simulink model "sedemo_event_translation_delay"  (Simulink 7.5)
settings: Solver=VariableStepDiscrete  StartTime=0.0  StopTime=20  MaxStep=0.2  RelTol=1e-3
libraries: simeventssink1 x3, simeventsqueue1 x1, simeventsgates1 x1, simeventstranslate1 x1, simeventsgenerators1 x1
settings Model: Creator=The MathWorks Inc.
settings OptimizationCC: InitFltsAndDblsToZero=on  EfficientMapNaN2IntZero=off
settings DebuggingCC: StrictBusMsg=Warning
settings SimEventsCC: propDiagAttribOutput=1  propDiagFcnCallOutput=1  propDiagStatOutput=0

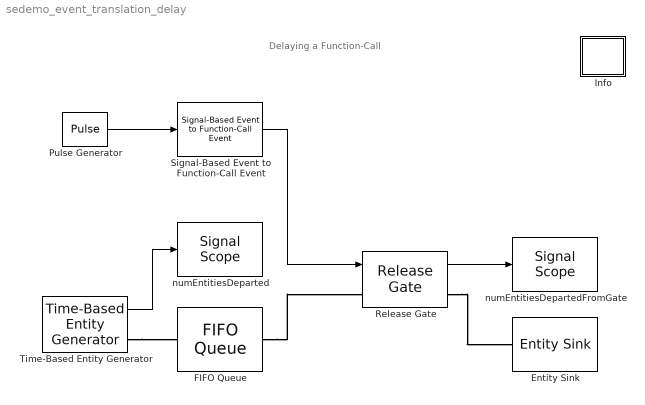
== system sedemo_event_translation_delay ==
  note: Delaying a Function-Call
  Entity Sink : simeventssink1/Entity Sink  Priority=1  SystemSampleTime=-1  AvailableForArrivals=on  StatNumberArrived=Off
  FIFO Queue : simeventsqueue1/FIFO Queue  Priority=1  SystemSampleTime=-1  Capacity=inf  EnableTOPort=off  StatNumberDeparted=Off  StatNumberInBlock=Off  StatPendingEntity=Off  StatAverageWait=Off  StatAverageQueueLength=Off  StatNumberTimedout=Off
      settings: AttributesFormatString=FIFO Queue Capacity =%<Capacity>
  Info : Subsystem
      settings: OpenFcn=simeventsdemohelp('sedemo_event_translation');
      mask Type: Info About This Model
      mask Help: evalc(['simeventsdemohelp(''sedemo_event_translation'');']);
      mask Display: disp('Info')
  Pulse Generator : DiscretePulseGenerator  PulseType=Time based  Amplitude=1  Period=5  PulseWidth=50  PhaseDelay=0  SampleTime=1
      settings: AttributesFormatString=Period = %<Period>\nPulse Width = %<PulseWidth>%
  Release Gate : simeventsgates1/Release Gate  Priority=1  SystemSampleTime=-1  OpenGateUpon=Function call from port fcn  SignalEdgeOption=Rising  SpecifyEventPriority=off  PriorityGateRelease=2200  StatNumberDeparted=On
  Signal-Based Event to Function-Call Event : simeventstranslate1/Signal-Based Event to Function-Call Event  Priority=1  SystemSampleTime=-1  GenerateFunctionCallUpon=Change in signal from port vc  SignalEdgeOption=Rising  EnableE1Port=off  EnableF2Port=off  EnableE2Port=off  SpecifyEventPriority=on  PriorityFunctionCall=200  FunctionCallDelayFrom=Dialog  DelayFunctionCall=2  StatNumberF1Calls=Off  StatNumberF2Calls=Off  MaskBlockType=none
      settings: AttributesFormatString=Function Call Delay = %<DelayFunctionCall>
  Time-Based Entity Generator : simeventsgenerators1/Entity Generators/Time-Based Entity Generator  Priority=1  DialogController=des_ddg_create  DialogControllerArgs=DataTag5  SystemSampleTime=-1  GenerateEntitiesUpon=Intergeneration time from dialog  Distribution=Constant  Minimum=0  Maximum=1  Mean=1  InitialSeed=12345  Period=5  PriorityEntityGeneration=300  GenerateEntityAtSimulationStart=on  ResponseWhenBlocked=Pause generation  ResponseWhenUnblocked=Immediate restart  EntityType=Blank  StatNumberDeparted=On  StatPendingEntity=Off  StatAverageIntergenerationTime=Off
      settings: AttributesFormatString=Distribution = %<Distribution>\nPeriod = %<Period>
  numEntitiesDeparted : simeventssink1/Signal Scope  Priority=1  SystemSampleTime=-1  PlotType=Stair  InputType=Signal  NumInputs=1  AttributeNameY=Count  XInputOptionSignal=Event time  XInputOptionEntity=Event time  AttributeNameX=Count  EnableEntityOutport=on  XMin=0  XMax=20  XLimitExceededOption=Stretch axis limits  YLimitExceededOption=Stretch axis limits  AxisGrid=on  AxisLegend=off  LineDisables=""  LineColors=b  LineStyles=-  LineMarkers=.  OpenScopeAtSimStart=on  Title=# of entities departed from Time-Based Generator  YLabel=""  XLabel=Time  FigurePosition=[311 436 318 217]  AxisZoom=off  DataStoreOption=Limited  DataPointsLimit=10000  StatNumberArrived=Off  ShowCountPlotted=off  ShowToolbar=on
      settings: YMin=0  YMax=10
  numEntitiesDepartedFromGate : simeventssink1/Signal Scope  Priority=1  SystemSampleTime=-1  PlotType=Stair  InputType=Signal  NumInputs=1  AttributeNameY=Count  XInputOptionSignal=Event time  XInputOptionEntity=Event time  AttributeNameX=Count  EnableEntityOutport=on  XMin=0  XMax=10  XLimitExceededOption=Stretch axis limits  YLimitExceededOption=Stretch axis limits  AxisGrid=on  AxisLegend=off  LineDisables=""  LineColors=b  LineStyles=-  LineMarkers=.  OpenScopeAtSimStart=on  Title=Number of Entities Served  YLabel=""  XLabel=Time  FigurePosition=[-7 439 312 214]  AxisZoom=off  DataStoreOption=Limited  DataPointsLimit=10000  StatNumberArrived=Off  ShowCountPlotted=off  ShowToolbar=on
      settings: YMin=0  YMax=10
  wires:
  Signal-Based Event to Function-Call Event/1 -> Release Gate/1
  Pulse Generator/1 -> Signal-Based Event to Function-Call Event/1
  Time-Based Entity Generator/1 -> numEntitiesDeparted/1
  Release Gate/1 -> numEntitiesDepartedFromGate/1
  connections:
  Time-Based Entity Generator/RConn1 -- FIFO Queue/LConn1
  FIFO Queue/RConn1 -- Release Gate/LConn1
  Release Gate/RConn1 -- Entity Sink/LConn1

== system sedemo_event_translation_delay/Info ==
